simulink model "Practica3"  (R2022b)
settings: Solver=VariableStepAuto  StartTime=0.0  StopTime=10  MaxStep=.0001  RelTol=1e-3
values from neighbouring files (symbols this model uses):
  b1 = 1000    [practica3.m]
  f = 0    [practica3.m]
  k1 = 16182    [practica3.m]
  k2 = 19000    [practica3.m]
  m1 = 290    [practica3.m]
  m2 = 59    [practica3.m]
libraries: simulink x1
settings Model: Creator=mluser  LastModifiedBy=mluser

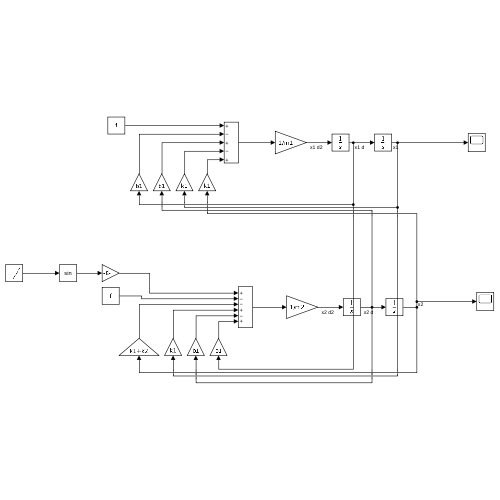
[thumbnail: Simulink's stored preview of the top-level diagram]
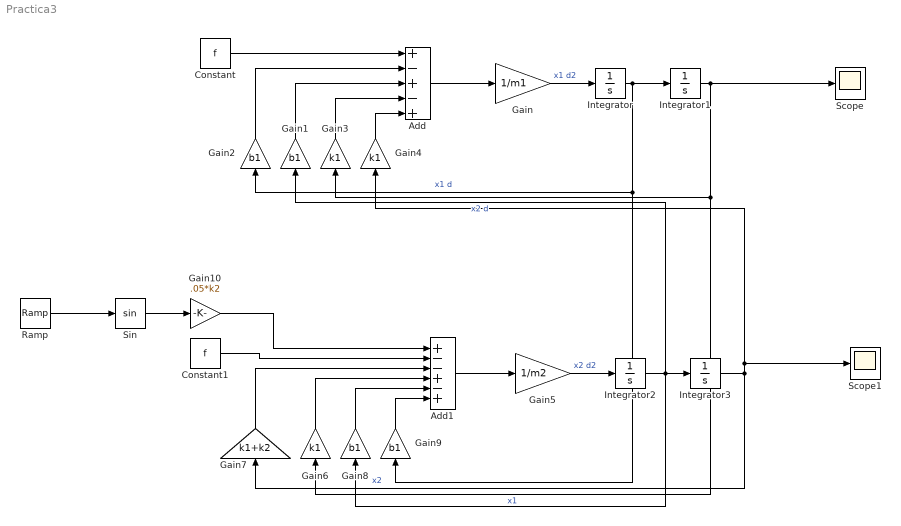
== system Practica3 ==
  Add : Sum  Inputs=+-+-+
  Add1 : Sum  Inputs=+--+-+
  Constant : Constant  Value=f
  Constant1 : Constant  Value=f
  Gain : Gain  Gain=1/m1
  Gain{1..2,8..9} (4 alike) : Gain  Gain=b1
  Gain10 : Gain  Gain=.05*k2
  Gain3 : Gain  Gain=k1
  Gain4 : Gain  Gain=k1
  Gain5 : Gain  Gain=1/m2
  Gain6 : Gain  Gain=k1
  Gain7 : Gain  Gain=k1+k2
  Integrator{,1..3} (4 alike) : Integrator
  Ramp : simulink/Sources/Ramp  slope=.5*pi  start=0  InitialOutput=0
  Scope : Scope
  Scope1 : Scope
  Sin : Trigonometry
  wires:
  Integrator/1 -> Gain9/1, Gain2/1, Integrator1/1  "x1 d"
  Gain/1 -> Integrator/1  "x1 d2"
  Add/1 -> Gain/1
  Integrator1/1 -> Scope/1, Gain3/1, Gain6/1  "x1"
  Constant/1 -> Add/1
  Gain4/1 -> Add/5
  Gain3/1 -> Add/4
  Gain1/1 -> Add/3
  Gain2/1 -> Add/2
  Gain9/1 -> Add1/6
  Gain6/1 -> Add1/4
  Gain7/1 -> Add1/3
  Constant1/1 -> Add1/2
  Add1/1 -> Gain5/1
  Gain8/1 -> Add1/5
  Gain5/1 -> Integrator2/1  "x2 d2"
  Integrator3/1 -> Scope1/1, Gain4/1, Gain7/1  "x2"
  Integrator2/1 -> Gain1/1, Gain8/1, Integrator3/1  "x2 d"
  Gain10/1 -> Add1/1
  Sin/1 -> Gain10/1
  Ramp/1 -> Sin/1
